simulink model "BMS"  (R2024a)
settings: Solver=ode23tb  StartTime=0.0  StopTime=500  RelTol=1e-3
undefined symbols (not defined in the file): Ion, Lithium
libraries: spsDiodeLib x11, spsIdealSwitchLib x10, spsBatteryLib x4, spsMosfetLib x2, spsSeriesRLCBranchLib x2, spsControlledCurrentSourceLib x1, spsDCVoltageSourceLib x1, fuzblock x1, spsPWMGenerator2LevelLib x1, spsSeriesRLCLoadLib x1, sps_lib x1
settings Model: SimulationMode=accelerator  Creator=Basnet  LastModifiedBy=Basnet
settings GRTTargetCC: RTWCAPISignals=on  RTWCAPIParams=on

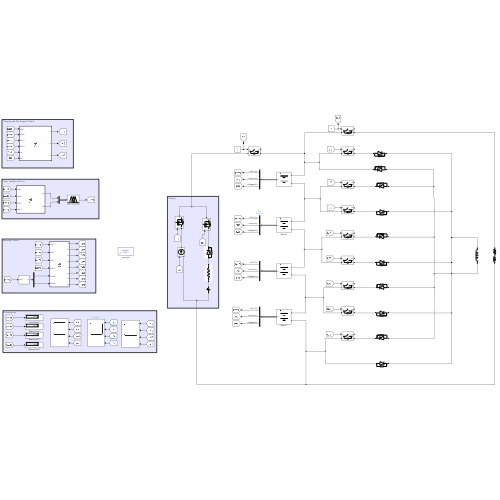
[thumbnail: Simulink's stored preview of the top-level diagram]
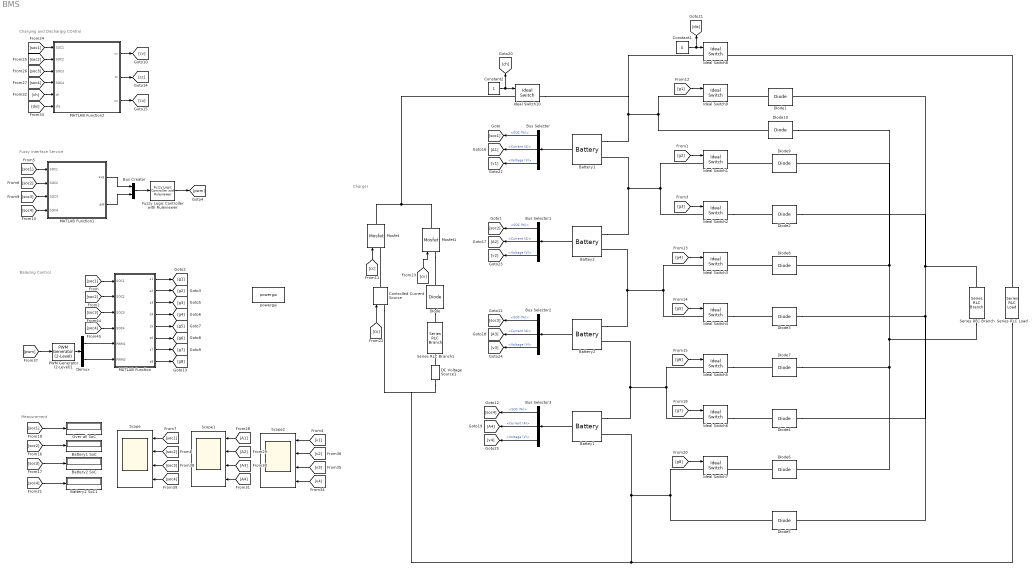
== system BMS ==
  note: Charger
  note: Balacing Control
  note: Charging and Dischargig COntrol
  note: Measurement
  note: Fuzzy Interface Service
  Battery1 : spsBatteryLib/Battery  BatType=Lithium-Ion  ShowTempParam=off  ThermalPreset=no  ShowAgeParam=off  NomV=3.7  NomQ=3  SOC=70  Batt_Tr=30  PresetModel=off  MaxQ=3  MinV=2.775  FullV=4.3068  Dis_rate=1.3043  R=0.012  Normal_OP=2.713  expZone="[3.9974     0.14739]"  current=[6.5 13 32.5]  Units=Time  Tci=20  NomT=20  T2=-30  MaxQ2=4.8  FullV2=7.1  Normal_OP2=5.655  expZone2="[6.58           1]"  Rca=0.6  ti=2000  Dp=0  Neq0=0  Tsim=1e6  Ta1=25  Qeol=5.4*0.9  Reol=0.013333*1.2  Char_age=[2.3478, 3]  Dis_age=[2.3478, 10]  N1=1500  N2=10500  N3=1000  N4=1400  Ta2=45  N5=950
  Battery1 SoC : Display
  Battery2 : spsBatteryLib/Battery  BatType=Lithium-Ion  ShowTempParam=off  ThermalPreset=no  ShowAgeParam=off  NomV=3.7  NomQ=3  SOC=66  Batt_Tr=30  PresetModel=off  MaxQ=3  MinV=2.775  FullV=4.3068  Dis_rate=1.3043  R=0.012  Normal_OP=2.713  expZone="[3.9974     0.14739]"  current=[6.5 13 32.5]  Units=Time  Tci=20  NomT=20  T2=-30  MaxQ2=4.8  FullV2=7.1  Normal_OP2=5.655  expZone2="[6.58           1]"  Rca=0.6  ti=2000  Dp=0  Neq0=0  Tsim=1e6  Ta1=25  Qeol=5.4*0.9  Reol=0.013333*1.2  Char_age=[2.3478, 3]  Dis_age=[2.3478, 10]  N1=1500  N2=10500  N3=1000  N4=1400  Ta2=45  N5=950
  Battery2 SoC : Display
  Battery2 SoC1 : Display
  Battey1 : spsBatteryLib/Battery  BatType=Lithium-Ion  ShowTempParam=off  ThermalPreset=no  ShowAgeParam=off  NomV=3.7  NomQ=3  SOC=64  Batt_Tr=30  PresetModel=off  MaxQ=3  MinV=2.775  FullV=4.3068  Dis_rate=1.3043  R=0.012  Normal_OP=2.713  expZone="[3.9974     0.14739]"  current=[6.5 13 32.5]  Units=Time  Tci=20  NomT=20  T2=-30  MaxQ2=4.8  FullV2=7.1  Normal_OP2=5.655  expZone2="[6.58           1]"  Rca=0.6  ti=2000  Dp=0  Neq0=0  Tsim=1e6  Ta1=25  Qeol=5.4*0.9  Reol=0.013333*1.2  Char_age=[2.3478, 3]  Dis_age=[2.3478, 10]  N1=1500  N2=10500  N3=1000  N4=1400  Ta2=45  N5=950
  Battey2 : spsBatteryLib/Battery  BatType=Lithium-Ion  ShowTempParam=off  ThermalPreset=no  ShowAgeParam=off  NomV=3.7  NomQ=3  SOC=68  Batt_Tr=30  PresetModel=off  MaxQ=3  MinV=2.775  FullV=4.3068  Dis_rate=1.3043  R=0.012  Normal_OP=2.713  expZone="[3.9974     0.14739]"  current=[6.5 13 32.5]  Units=Time  Tci=20  NomT=20  T2=-30  MaxQ2=4.8  FullV2=7.1  Normal_OP2=5.655  expZone2="[6.58           1]"  Rca=0.6  ti=2000  Dp=0  Neq0=0  Tsim=1e6  Ta1=25  Qeol=5.4*0.9  Reol=0.013333*1.2  Char_age=[2.3478, 3]  Dis_age=[2.3478, 10]  N1=1500  N2=10500  N3=1000  N4=1400  Ta2=45  N5=950
  Bus Creator : BusCreator  Inputs=2
  Bus Selector{,1..3} (4 alike) : BusSelector  OutputSignals=SOC (%),Current (A),Voltage (V)
  Constant1 : Constant  Value=0
  Constant2 : Constant
  Controlled Current Source : spsControlledCurrentSourceLib/Controlled Current Source  Initialize=on  Source_Type=AC  Amplitude=0  Phase=0  Frequency=0  Measurements=None
  DC Voltage Source1 : spsDCVoltageSourceLib/DC Voltage Source  Amplitude=18  Measurements=None
  Demux : Demux  Outputs=2
  Diode{,1..10} (11 alike) : spsDiodeLib/Diode  Ron=0.001  Lon=0  Vf=0.8  IC=0  UseSnubber=0  Rs=500  Cs=250e-9  Measurements=off
  Fuzzy Logic Controller with Ruleviewer : fuzblock/Fuzzy Logic  Controller  with Ruleviewer  fismatrix=group  Ts=2
  Ideal Switch{1..10} (10 alike) : spsIdealSwitchLib/Ideal Switch  Ron=0.001  Lon=0  IC=0  Rs=1e5  Cs=inf  Measurements=on
  MATLAB Function : MATLAB Function  TreatAsAtomicUnit=on
  MATLAB Function1 : MATLAB Function  TreatAsAtomicUnit=on
  MATLAB Function2 : MATLAB Function  TreatAsAtomicUnit=on
  Mosfet : spsMosfetLib/Mosfet  Ron=0.1  Lon=0  Rd=0.01  Vfd=0  IC=0  Rs=1e5  Cs=inf  Measurements=off
  Mosfet1 : spsMosfetLib/Mosfet  Ron=0.1  Lon=0  Rd=0.01  Vfd=0  IC=0  Rs=1e5  Cs=inf  Measurements=off
  Over all SoC : Display
  PWM Generator (2-Level)1 : spsPWMGenerator2LevelLib/PWM Generator (2-Level)  ModulatorType=Single-phase half-bridge (2 pulses)  ModulatorMode=Unsynchronized  Fc=5000  Pc=90  nF=27  MinMax="[ 0  1 ]"  SamplingTechnique=Natural  ModulatingSignals=off  m=0.8  Freq=60  Phase=0  Ts=0.00001  ShowCarrierOutport=off
  Scope : Scope  NumInputPorts=4
  Scope1 : Scope  NumInputPorts=4
  Scope2 : Scope  NumInputPorts=4
  Series RLC Branch : spsSeriesRLCBranchLib/Series RLC Branch  LConnTagsString=__new0  RConnTagsString=__new0  BranchType=L  Resistance=0.05  Inductance=1.5e-3  SetiL0=off  InitialCurrent=0  Capacitance=1e-6  Setx0=off  InitialVoltage=0  Measurements=None
  Series RLC Branch1 : spsSeriesRLCBranchLib/Series RLC Branch  LConnTagsString=__new0  RConnTagsString=__new0  BranchType=R  Resistance=0.1  Inductance=1e-3  SetiL0=off  InitialCurrent=0  Capacitance=1e-6  Setx0=off  InitialVoltage=0  Measurements=None
  Series RLC Load : spsSeriesRLCLoadLib/Series RLC Load  LConnTagsString=a  RConnTagsString=__new0  NominalVoltage=15  NominalFrequency=60  ActivePower=10  InductivePower=5  CapacitivePower=0  Setx0=off  InitialVoltage=0  SetiL0=off  InitialCurrent=0  Measurements=Branch current  LoadType=constant Z
  powergui : sps_lib/powergui  Priority=1  SimulationMode=Discrete  SampleTime=0.00005  frequency=60  Iterations=50  frequencyindice=0  Pbase=100e6  ErrMax=1e-4  UnitsV=kV  UnitsW=MW  buscounter=0  FunctionMessages=off  echomessages=off  EnableUseOfTLC=off  CurrentSourceSwitches=off  DisableSnubberDevices=off  DisableRonSwitches=off  DisableVfSwitches=off  DisplayEquations=off  AutomaticDiscreteSolvers=off  SolverType=Tustin/Backward Euler (TBE)  Interpol=off  ExternalGateDelay=off  methode=off  Ts=100  x0status=blocks  SPID=on  SwTol=0  HookPort=off  NonlinearTolerance=1e-4  nMaxIteration=100  ContinueOnMaxIteration=off  RestoreLinks=warning  ResistiveCurrentMeasurement=off  Frange=[0:2:500]  Ylog=off  Xlog=on  ShowGrid=off  save=off  variable=ZData  structure=0  ZoomFFT=off  StartTime=0.0  cycles=1  DisplayStyle=1  fundamental=60  FreqAxis=off  MaxFrequency=1000  frequencyindicesteady=1  RmsSteady=1  display=off
  wires:
  [soc3] -> Scope/3
  Battery2/1 -> Bus Selector2/1
  [soc4] -> Scope/4
  [soc2] -> Scope/2
  Battey1/1 -> Bus Selector3/1
  Battery1/1 -> Bus Selector/1
  [soc1] -> Over all SoC/1
  Bus Selector/1 -> [soc1]  "<SOC (%)>"
  [soc3] -> Battery2 SoC/1
  Bus Selector2/1 -> [soc3]  "<SOC (%)>"
  [soc1] -> Scope/1
  Battey2/1 -> Bus Selector1/1
  [soc2] -> Battery1 SoC/1
  Bus Selector3/1 -> [soc4]  "<SOC (%)>"
  Bus Selector1/1 -> [soc2]  "<SOC (%)>"
  PWM Generator (2-Level)1/1 -> Demux/1
  Demux/1 -> MATLAB Function/5(PWM1)
  [soc1] -> MATLAB Function/1(SOC1)
  [soc2] -> MATLAB Function/2(SOC2)
  MATLAB Function/1(s1) -> [g1]
  MATLAB Function/2(s2) -> [g2]
  MATLAB Function/3(s3) -> [g3]
  MATLAB Function/5(s5) -> [g5]
  MATLAB Function/6(s6) -> [g6]
  MATLAB Function/4(s4) -> [g4]
  [g1] -> Ideal Switch9/1
  [g3] -> Ideal Switch2/1
  [g4] -> Ideal Switch3/1
  Demux/2 -> MATLAB Function/6(PWM2)
  [soc3] -> MATLAB Function/3(SOC3)
  [soc4] -> MATLAB Function/4(SOC4)
  MATLAB Function/7(s7) -> [g7]
  MATLAB Function/8(s8) -> [g8]
  [g8] -> Ideal Switch7/1
  [g7] -> Ideal Switch6/1
  [g6] -> Ideal Switch5/1
  [g5] -> Ideal Switch4/1
  [g2] -> Ideal Switch1/1
  [soc4] -> Battery2 SoC1/1
  Constant1/1 -> [dis], Ideal Switch8/1
  Constant2/1 -> [ch], Ideal Switch10/1
  Fuzzy Logic Controller with Ruleviewer/1 -> [pwm]
  MATLAB Function1/1(avg) -> Bus Creator/1
  MATLAB Function1/2(diff) -> Bus Creator/2
  [soc1] -> MATLAB Function1/1(SOC1)
  [soc2] -> MATLAB Function1/2(SOC2)
  [soc3] -> MATLAB Function1/3(SOC3)
  [soc4] -> MATLAB Function1/4(SOC4)
  Bus Creator/1 -> Fuzzy Logic Controller with Ruleviewer/1
  [cc] -> Mosfet/1
  [cu] -> Controlled Current Source/1
  [cv] -> Mosfet1/1
  [soc1] -> MATLAB Function2/1(SOC1)
  [soc2] -> MATLAB Function2/2(SOC2)
  [soc3] -> MATLAB Function2/3(SOC3)
  [soc4] -> MATLAB Function2/4(SOC4)
  MATLAB Function2/3(cu) -> [cu]
  MATLAB Function2/2(cc) -> [cc]
  MATLAB Function2/1(cv) -> [cv]
  [A1] -> Scope1/1
  [A2] -> Scope1/2
  [A3] -> Scope1/3
  [A4] -> Scope1/4
  Bus Selector/2 -> [A1]  "<Current (A)>"
  Bus Selector1/2 -> [A2]  "<Current (A)>"
  Bus Selector2/2 -> [A3]  "<Current (A)>"
  Bus Selector3/2 -> [A4]  "<Current (A)>"
  [ch] -> MATLAB Function2/5(ch)
  [dis] -> MATLAB Function2/6(dis)
  [pwm] -> PWM Generator (2-Level)1/1
  [v1] -> Scope2/1
  Bus Selector/3 -> [v1]  "<Voltage (V)>"
  Bus Selector1/3 -> [v2]  "<Voltage (V)>"
  Bus Selector2/3 -> [v3]  "<Voltage (V)>"
  Bus Selector3/3 -> [v4]  "<Voltage (V)>"
  [v4] -> Scope2/4
  [v2] -> Scope2/2
  [v3] -> Scope2/3
  connections:
  Ideal Switch2/LConn1 -- Ideal Switch1/LConn1 -- Battery1/LConn2 -- Battey2/LConn1
  Ideal Switch4/LConn1 -- Ideal Switch3/LConn1 -- Battey2/LConn2 -- Battery2/LConn1
  Series RLC Branch/LConn1 -- Diode2/RConn1 -- Diode1/RConn1 -- Diode5/RConn1 -- Diode4/RConn1 -- Diode3/RConn1
  Ideal Switch6/LConn1 -- Battery2/LConn2 -- Battey1/LConn1 -- Ideal Switch5/LConn1
  Diode1/LConn1 -- Ideal Switch9/RConn1
  Series RLC Branch/RConn1 -- Diode10/LConn1 -- Diode9/LConn1 -- Diode8/LConn1 -- Diode6/LConn1 -- Diode7/LConn1
  Ideal Switch2/RConn1 -- Diode2/LConn1
  Ideal Switch4/RConn1 -- Diode3/LConn1
  Ideal Switch6/RConn1 -- Diode4/LConn1
  Diode5/LConn1 -- Battey1/LConn2 -- Controlled Current Source/LConn1 -- DC Voltage Source1/LConn1 -- Series RLC Load/RConn1 -- Ideal Switch7/LConn1
  Diode6/RConn1 -- Ideal Switch7/RConn1
  Ideal Switch5/RConn1 -- Diode7/RConn1
  Diode8/RConn1 -- Ideal Switch3/RConn1
  Diode9/RConn1 -- Ideal Switch1/RConn1
  Battery1/LConn1 -- Ideal Switch10/RConn1 -- Ideal Switch8/LConn1 -- Diode10/RConn1 -- Ideal Switch9/LConn1
  Series RLC Load/LConn1 -- Ideal Switch8/RConn1
  Mosfet/RConn1 -- Ideal Switch10/LConn1 -- Mosfet1/RConn1
  Controlled Current Source/RConn1 -- Mosfet/LConn1
  Mosfet1/LConn1 -- Diode/RConn1
  Diode/LConn1 -- Series RLC Branch1/LConn1
  DC Voltage Source1/RConn1 -- Series RLC Branch1/RConn1

== matlab function BMS/MATLAB Function1 ==
  data: SOC1 input; avg output; SOC2 input; SOC3 input; SOC4 input; diff output
function [avg, diff] = fcn(SOC1,SOC2,SOC3,SOC4)
High = max([SOC1 SOC2 SOC3 SOC4]);
Low = min([SOC1 SOC2 SOC3 SOC4]);
if High==SOC1&&Low==SOC2
    avg=(SOC1+SOC2)*0.5;
    diff=SOC1-SOC2;
elseif High==SOC1&&Low==SOC3
    avg=(SOC1+SOC3)*0.5;
    diff=SOC1-SOC3;
elseif High==SOC1&&Low==SOC4
    avg=(SOC1+SOC4)*0.5;
    diff=SOC1-SOC4;
elseif High==SOC2&&Low==SOC1
    avg=(SOC2+SOC1)*0.5;
    diff=SOC2-SOC1;
elseif High==SOC2&&Low==SOC3
    avg=(SOC2+SOC3)*0.5;
    diff=SOC2-SOC3;
elseif High==SOC2&&Low==SOC4
    avg=(SOC2+SOC4)*0.5;
    diff=SOC2-SOC4;
elseif High==SOC3&&Low==SOC1
    avg=(SOC3+SOC1)*0.5;
    diff=SOC3-SOC1;
elseif High==SOC3&&Low==SOC2
    avg=(SOC3+SOC2)*0.5;
    diff=SOC3-SOC2;
elseif High==SOC3&&Low==SOC4
    avg=(SOC3+SOC4)*0.5;
    diff=SOC3-SOC4;
elseif High==SOC4&&Low==SOC1
    avg=(SOC4+SOC1)*0.5;
    diff=SOC4-SOC1;
elseif High==SOC4&&Low==SOC2
    avg=(SOC4+SOC2)*0.5;
    diff=SOC4-SOC2;
elseif High==SOC4&&Low==SOC3
    avg=(SOC4+SOC3)*0.5;
    diff=SOC4-SOC3;
else
    avg=0;
    diff=0;
end
end

== matlab function BMS/MATLAB Function ==
  data: s1 output; SOC1 input; SOC2 input; SOC3 input; s2 output; s3 output; s4 output; s5 output; s6 output; SOC4 input; PWM1 input; PWM2 input; s7 output; s8 output
function [s1,s2,s3,s4,s5,s6,s7,s8] = fcn(SOC1,SOC2,SOC3,SOC4,PWM1,PWM2)
High = max([SOC1 SOC2 SOC3 SOC4]);
Low = min([SOC1 SOC2 SOC3 SOC4]);
if High==SOC1&&Low==SOC2
    s1=PWM1; s2=1; s5=PWM2;
    s3=0; s4=0; s6=0; s7=0; s8=0;
elseif High==SOC1&&Low==SOC3
    s1=PWM1; s2=PWM1; s4=PWM2; s7=PWM2;
    s3=0; s5=0; s6=0; s8=0;
elseif High==SOC1&&Low==SOC4
    s1=PWM1; s2=PWM1; s6=PWM2;
    s3=0; s4=0; s5=0; s7=0; s8=0;
elseif High==SOC2&&Low==SOC1
    s3=1; s4=PWM1;
    s1=0; s2=0; s5=0; s6=0; s7=0; s8=0;
elseif High==SOC2&&Low==SOC3
    s3=PWM1; s4=1; s7=PWM2;
    s1=0; s2=0; s5=0; s6=0; s8=0;
elseif High==SOC2&&Low==SOC4
    s3=PWM1; s4=PWM1; s6=PWM2;
    s1=0; s2=0; s5=0; s7=0; s8=0;
elseif High==SOC3&&Low==SOC1
    s3=PWM2; s5=PWM1; s6=PWM1;
    s1=0; s2=0; s4=0; s7=0; s8=0;
elseif High==SOC3&&Low==SOC2
    s2=PWM2; s5=1; s6=PWM1;
    s1=0; s3=0; s4=0; s7=0; s8=0;
elseif High==SOC3&&Low==SOC4
    s5=PWM1; s6=1;
    s1=0; s2=0; s3=0; s4=0; s7=0; s8=0;
elseif High==SOC4&&Low==SOC1
    s3=PWM2; s7=PWM1; s8=PWM1;
    s1=0; s2=0; s4=0; s5=0; s6=0;
elseif High==SOC4&&Low==SOC2
    s2=PWM2; s5=PWM2; s7=PWM1; s8=PWM1;
    s1=0; s3=0; s4=0; s6=0;
elseif High==SOC4&&Low==SOC3
    s4=PWM2; s8=PWM1; s7=1;
    s1=0; s2=0; s3=0; s5=0; s6=0;
else
    s1=0; s2=0; s3=0; s4=0; s5=0; s6=0; s7=0; s8=0;
end
end

== matlab function BMS/MATLAB Function2 ==
  data: SOC1 input; SOC2 input; SOC3 input; SOC4 input; cv output; cc output; cu output; ch input; dis input
function [cv, cc, cu] = fcn(SOC1, SOC2, SOC3, SOC4, ch, dis)
cv=0; 
cc=0;
cu=0;
socavg=(SOC1+SOC2+SOC3+SOC4)*0.25;
if ((ch==1) && (dis==0))
if(socavg<80)
    cu=10;
    cc=1;
    cv=0;
elseif(socavg>=80)
    cu=0;
    cc=0;
    cv=1;
else(socavg==100)
    cu=0;
    cc=0;
    cv=0;
end
elseif ((ch==0) && (dis==1))
    cu=0;
    cc=0;
    cv=0;
end
